simulink model "F16"  (R2024a)
settings: configuration reference "standardSILConfiguraitonParams" (kept outside this file)
undefined symbols (not defined in the file): actuatorDelay_s, plantSampleTime_s
settings Model: Creator=GTAR  LastModifiedBy=jerem
settings ConfigSetRef: SourceName=standardSILConfiguraitonParams  SourceLocation=Base Workspace

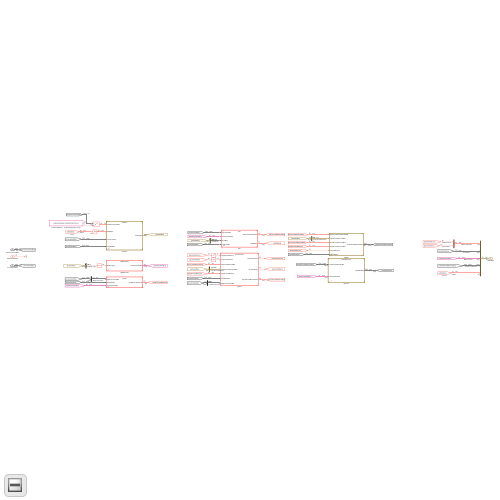
[thumbnail: Simulink's stored preview of the top-level diagram]
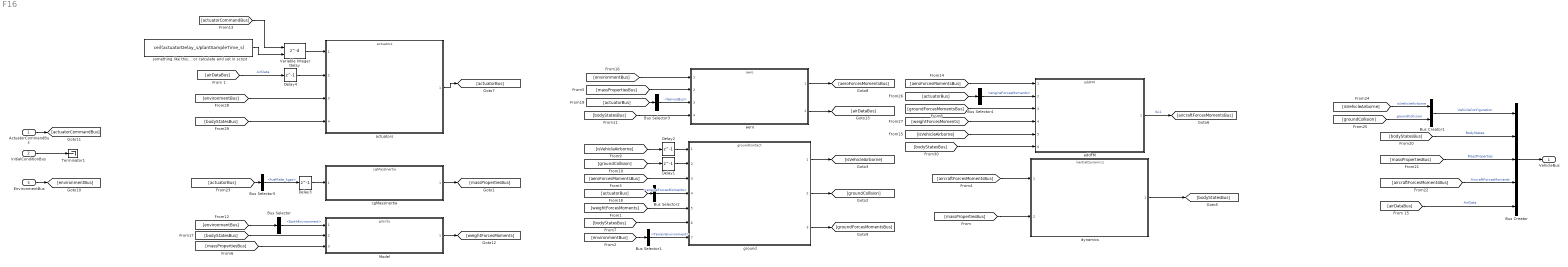
== system F16 ==
  ActuatorCommandBus : Inport  OutDataTypeStr=Bus: ActuatorCommandBus
  InitialConditionBus : Inport  Port=2
  EnvironmentBus : Inport  Port=3  OutDataTypeStr=Bus: EnvironmentBus
  Bus Creator : BusCreator  Inputs=5  OutDataTypeStr=Bus: VehicleBus
  Bus Creator1 : BusCreator  Inputs=2  OutDataTypeStr=Bus: VehicleConfigurationBus
  Bus Selector : BusSelector  OutputSignals=EarthEnvironment
  Bus Selector1 : BusSelector  OutputSignals=TerrainEnvironment
  Bus Selector2 : BusSelector  OutputSignals=EngineBus.engineForcesMoments
  Bus Selector3 : BusSelector  OutputSignals=ServosBus
  Bus Selector4 : BusSelector  OutputSignals=EngineBus.engineForcesMoments
  Bus Selector5 : BusSelector  OutputSignals=EngineBus.fuelRate_kgps
  Delay{1..4} (4 alike) : Delay  DelayLength=1  InitialCondition=0
  Model : ModelReference  ModelNameDialog=gravity.slx  SimulationMode=Normal  ModelReferenceVersion=1.26
  Terminator1 : Terminator
  Variable Integer Delay : Delay  DelayLengthSource=Input port
      settings: InputPortMap=u0,p1
  actuators : ModelReference  ModelNameDialog=actuators.slx  SimulationMode=Normal  ModelReferenceVersion=1.83
  addFM : ModelReference  ModelNameDialog=addFM.slx  SimulationMode=Normal  ModelReferenceVersion=1.68
  aero : ModelReference  ModelNameDialog=aero.slx  SimulationMode=Normal  ModelReferenceVersion=1.297
  cgMassInertia : ModelReference  ModelNameDialog=cgMassInertia.slx  SimulationMode=Normal  ModelReferenceVersion=1.42
  dynamics : ModelReference  ModelNameDialog=inertialDynamics.slx  SimulationMode=Normal  ModelReferenceVersion=1.34
  ground : ModelReference  ModelNameDialog=groundContact.slx  SimulationMode=Normal  ModelReferenceVersion=1.95
  something like this... or calculate and set in script : Constant  Value=ceil(actuatorDelay_s/plantSampleTime_s)
  VehicleBus : Outport  OutDataTypeStr=Bus: VehicleBus
  wires:
  actuators/1 -> [actuatorBus]
  something like this... or calculate and set in script/1 -> Variable Integer Delay/2
  InitialConditionBus/1 -> Terminator1/1
  Bus Selector3/1 -> aero/3  "<ServosBus>"
  [massPropertiesBus] -> dynamics/2
  [massPropertiesBus] -> aero/2
  Bus Creator/1 -> VehicleBus/1
  Variable Integer Delay/1 -> actuators/1
  addFM/1 -> [aircraftForcesMomentsBus]  "6x1"
  aero/1 -> [aeroForcesMomentsBus]
  [bodyStatesBus] -> aero/4
  EnvironmentBus/1 -> [environmentBus]
  ActuatorCommandBus/1 -> [actuatorCommandBus]
  [actuatorCommandBus] -> Variable Integer Delay/1
  [aeroForcesMomentsBus] -> addFM/1
  [environmentBus] -> aero/1
  Model/1 -> [weightForcesMoments]
  Bus Selector4/1 -> addFM/2  "<engineForcesMoments>"
  [groundForcesMomentsBus] -> addFM/3
  ground/3 -> [groundForcesMomentsBus]
  cgMassInertia/1 -> [massPropertiesBus]
  [weightForcesMoments] -> ground/5
  [aeroForcesMomentsBus] -> ground/3
  [bodyStatesBus] -> ground/6
  ground/1 -> [isVehicleAirborne]
  ground/2 -> [groundCollision]
  Delay2/1 -> ground/1
  Delay1/1 -> ground/2
  [isVehicleAirborne] -> Delay2/1
  [groundCollision] -> Delay1/1
  [massPropertiesBus] -> Model/3
  [environmentBus] -> Bus Selector/1
  Bus Selector/1 -> Model/1  "<EarthEnvironment>"
  [bodyStatesBus] -> Model/2
  [environmentBus] -> Bus Selector1/1
  [actuatorBus] -> Bus Selector2/1
  [actuatorBus] -> Bus Selector3/1
  Bus Selector2/1 -> ground/4  "<engineForcesMoments>"
  [bodyStatesBus] -> Bus Creator/2  "BodyStates"
  [massPropertiesBus] -> Bus Creator/3  "MassProperties"
  [aircraftForcesMomentsBus] -> Bus Creator/4  "AircraftForcesMoments"
  Bus Creator1/1 -> Bus Creator/1  "VehicleConfiguration"
  [groundCollision] -> Bus Creator1/2  "groundCollision"
  [isVehicleAirborne] -> Bus Creator1/1  "isVehicleAirborne"
  [actuatorBus] -> Bus Selector4/1
  dynamics/1 -> [bodyStatesBus]
  Bus Selector1/1 -> ground/7  "<TerrainEnvironment>"
  aero/2 -> [airDataBus]
  [airDataBus] -> Bus Creator/5  "AirData"
  [aircraftForcesMomentsBus] -> dynamics/1
  [actuatorBus] -> Bus Selector5/1
  Bus Selector5/1 -> Delay3/1  "<fuelRate_kgps>"
  Delay3/1 -> cgMassInertia/1
  [weightForcesMoments] -> addFM/4
  [airDataBus] -> Delay4/1  "AirData"
  [environmentBus] -> actuators/3
  [bodyStatesBus] -> actuators/4
  Delay4/1 -> actuators/2
  [isVehicleAirborne] -> addFM/5
  [bodyStatesBus] -> addFM/6
